simulink model "FSMK_DRC"  (R2015a)
settings: Solver=ode5  StartTime=0.0  StopTime=20  FixedStep=dt  RelTol=1e-3
values from neighbouring files (symbols this model uses):
  A = [0 -87.2734439167 0 0 0 0 87.2734439167 -1.74546887833 0 0 0 0 ... (36 elements, 6x6)]    [A.mat]    (also in A_decompose.m = 0.01*[-0.773996386153021,96.9795539479971,0,0,0,0;-96.400970)
  A_real = A+M_A*N_A*10    [controller.m]
  B = [0  0; 43537  27917; 0  0; 192690  -42273; 0  0; -338240  439030]    [B.mat]    (also in B_decompose.m = 0.01*[-0.230745598618469,-0.153904745996477;0.06127775595526)
  B_real = B+M_B*N_B*10    [controller.m]
  C = [0 -5.1012 0 4.026 0 3.2726]    [C.mat]    (also in C_decompose.m = 0.01*[-23.1554338545303,9.56281796834669,0.435674513053965,-)
  C_real = C+M_C*N_C*10    [controller.m]
  dt = 1e-3    (= 0.001)    [controller.m]
  H = [0 -5.4265 0 5.0795 0 5.0035]    [H.mat]
  Lk = [-59.477792404 31.7484157566 3951.54702126 -4057.82953256 6373.12577438 -2161.86440143]    [Lk.mat]
  Ls = -Ls*1.5e13    [controller.m]
  max_derror = 5    [controller.m]
  max_error = 0.01    [controller.m]
undefined symbols (not defined in the file or in its folder): K
libraries: simulink x2, fuzblock x1
settings Model: Creator=p4wp4w  LastModifiedBy=p4wp4w

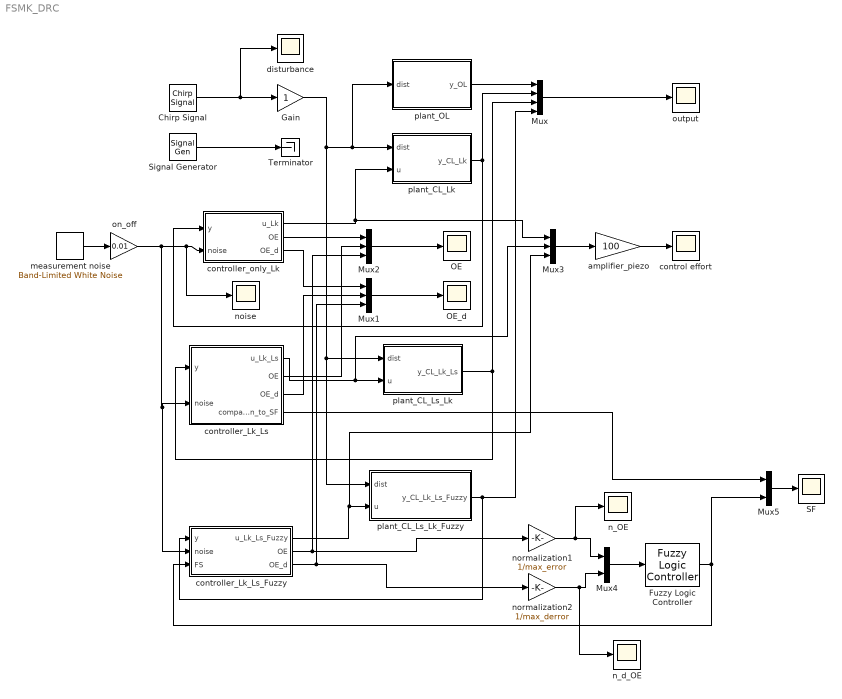
== system FSMK_DRC ==
  Chirp Signal : simulink/Sources/Chirp Signal  f1=0.1  T=20  f2=100
  Fuzzy Logic Controller : fuzblock/Fuzzy Logic  Controller  fis='FSMO.fis'
  Gain : Gain
  Mux : Mux
  Mux1 : Mux  Inputs=3
  Mux2 : Mux  Inputs=3
  Mux3 : Mux  Inputs=3
  Mux4 : Mux  Inputs=2
  Mux5 : Mux  Inputs=2
  OE : Scope
      settings: ShowLegends=on  YMin=-0.01  YMax=0.01  SaveName=OE
  OE_d : Scope
      settings: ShowLegends=on  YMin=-3.5  YMax=3.5  SaveName=d_OE
  SF : Scope
      settings: ShowLegends=on  YMin=-1  YMax=1  SaveName=SF
  Signal Generator : SignalGenerator  WaveForm=square  Frequency=1/5
  Terminator : Terminator
  amplifier_piezo : Gain  Gain=100
  control effort : Scope
      settings: ShowLegends=on  YMin=-50  YMax=50  SaveName=control_effort
  controller_Lk_Ls : Subsystem
  controller_Lk_Ls_Fuzzy : Subsystem
  controller_only_Lk : Subsystem
  disturbance : Scope
      settings: ShowLegends=on  YMin=-1.5  YMax=1.5  SaveName=disturbance
  measurement noise : simulink/Sources/Band-Limited White Noise  Cov=[0.000000001]  Ts=dt  seed=[23341]
  n_OE : Scope
      settings: ShowLegends=on  YMin=-1  YMax=1  SaveName=n_OE
  n_d_OE : Scope
      settings: ShowLegends=on  YMin=-0.8  YMax=0.7  SaveName=n_d_OE
  noise : Scope
      settings: SaveName=ScopeData2
  normalization1 : Gain  Gain=1/max_error
  normalization2 : Gain  Gain=1/max_derror
  on_off : Gain  Gain=0.01
  output : Scope
      settings: ShowLegends=on  YMin=-0.25  YMax=0.25  SaveName=output
  plant_CL_Lk : Subsystem
  plant_CL_Ls_Lk : Subsystem
  plant_CL_Ls_Lk_Fuzzy : Subsystem
  plant_OL : Subsystem
  wires:
  plant_CL_Lk/1(y_CL_Lk) -> controller_only_Lk/1(y), Mux/2
  plant_OL/1(y_OL) -> Mux/1
  controller_only_Lk/1(u_Lk) -> Mux3/1, plant_CL_Lk/2(u)
  measurement noise/1 -> on_off/1
  controller_Lk_Ls/1(u_Lk_Ls) -> Mux3/2, plant_CL_Ls_Lk/2(u)
  controller_only_Lk/3(OE_d) -> Mux1/1
  controller_only_Lk/2(OE) -> Mux2/1
  controller_Lk_Ls/2(OE) -> Mux2/2
  controller_Lk_Ls/3(OE_d) -> Mux1/2
  on_off/1 -> controller_Lk_Ls_Fuzzy/2(noise), controller_Lk_Ls/2(noise), noise/1, controller_only_Lk/2(noise)
  plant_CL_Ls_Lk/1(y_CL_Lk_Ls) -> Mux/3, controller_Lk_Ls/1(y)
  Mux3/1 -> amplifier_piezo/1
  controller_Lk_Ls_Fuzzy/1(u_Lk_Ls_Fuzzy) -> Mux3/3, plant_CL_Ls_Lk_Fuzzy/2(u)
  plant_CL_Ls_Lk_Fuzzy/1(y_CL_Lk_Ls_Fuzzy) -> controller_Lk_Ls_Fuzzy/1(y), Mux/4
  controller_Lk_Ls_Fuzzy/2(OE) -> Mux2/3, normalization1/1
  controller_Lk_Ls_Fuzzy/3(OE_d) -> Mux1/3, normalization2/1
  normalization1/1 -> n_OE/1, Mux4/1
  normalization2/1 -> n_d_OE/1, Mux4/2
  Mux4/1 -> Fuzzy Logic Controller/1
  Fuzzy Logic Controller/1 -> controller_Lk_Ls_Fuzzy/3(FS), Mux5/2
  controller_Lk_Ls/4(comparison_to_SF) -> Mux5/1
  Mux5/1 -> SF/1
  Gain/1 -> plant_CL_Ls_Lk_Fuzzy/1(dist), plant_CL_Ls_Lk/1(dist), plant_OL/1(dist), plant_CL_Lk/1(dist)
  amplifier_piezo/1 -> control effort/1
  Mux/1 -> output/1
  Mux2/1 -> OE/1
  Mux1/1 -> OE_d/1
  Chirp Signal/1 -> disturbance/1, Gain/1
  Signal Generator/1 -> Terminator/1

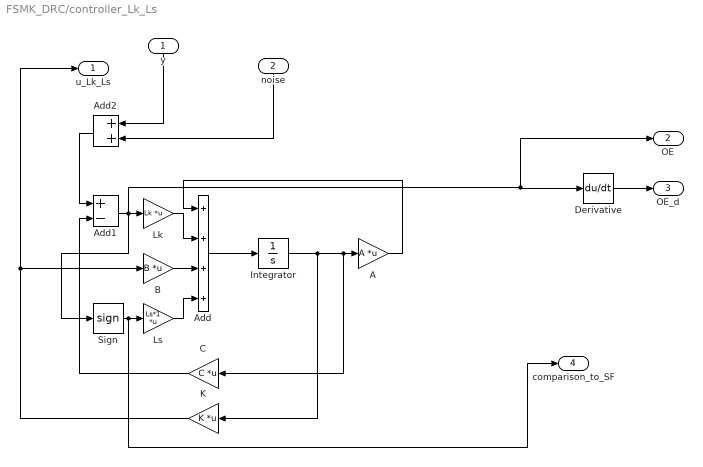
== system FSMK_DRC/controller_Lk_Ls ==
  y : Inport
  noise : Inport  Port=2
  A : Gain  Gain=A  Multiplication=Matrix(K*u)
  Add : Sum  Inputs=++++
  Add1 : Sum  Inputs=+-
  Add2 : Sum
  B : Gain  Gain=B  Multiplication=Matrix(K*u)
  C : Gain  Gain=C  Multiplication=Matrix(K*u)
  Derivative : Derivative
  Integrator : Integrator
  K : Gain  Gain=K  Multiplication=Matrix(K*u)
  Lk : Gain  Gain=Lk  Multiplication=Matrix(K*u)
  Ls : Gain  Gain=Ls*1  Multiplication=Matrix(K*u)
  Sign : Signum
  u_Lk_Ls : Outport
  OE : Outport  Port=2
  OE_d : Outport  Port=3
  comparison_to_SF : Outport  Port=4
  wires:
  Derivative/1 -> OE_d/1
  noise/1 -> Add2/2
  Add1/1 -> Sign/1, Lk/1, OE/1, Derivative/1
  C/1 -> Add1/2
  Add/1 -> Integrator/1
  Add2/1 -> Add1/1
  Lk/1 -> Add/2
  A/1 -> Add/1
  B/1 -> Add/3
  Integrator/1 -> A/1, C/1, K/1
  K/1 -> B/1, u_Lk_Ls/1
  y/1 -> Add2/1
  Ls/1 -> Add/4
  Sign/1 -> comparison_to_SF/1, Ls/1

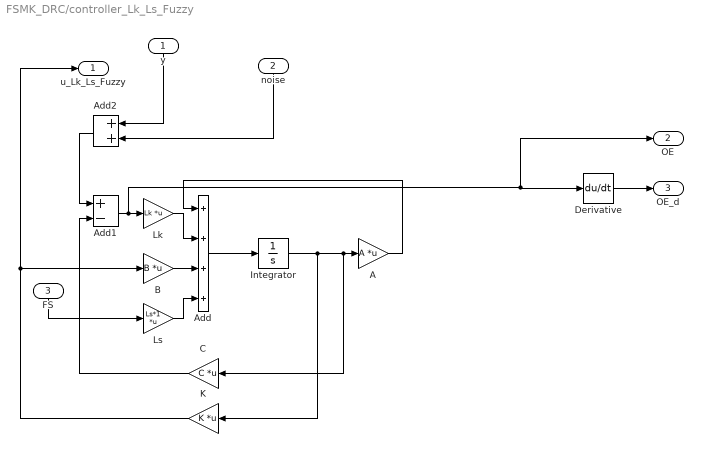
== system FSMK_DRC/controller_Lk_Ls_Fuzzy ==
  y : Inport
  noise : Inport  Port=2
  FS : Inport  Port=3
  A : Gain  Gain=A  Multiplication=Matrix(K*u)
  Add : Sum  Inputs=++++
  Add1 : Sum  Inputs=+-
  Add2 : Sum
  B : Gain  Gain=B  Multiplication=Matrix(K*u)
  C : Gain  Gain=C  Multiplication=Matrix(K*u)
  Derivative : Derivative
  Integrator : Integrator
  K : Gain  Gain=K  Multiplication=Matrix(K*u)
  Lk : Gain  Gain=Lk  Multiplication=Matrix(K*u)
  Ls : Gain  Gain=Ls*1  Multiplication=Matrix(K*u)
  u_Lk_Ls_Fuzzy : Outport
  OE : Outport  Port=2
  OE_d : Outport  Port=3
  wires:
  FS/1 -> Ls/1
  Ls/1 -> Add/4
  y/1 -> Add2/1
  K/1 -> u_Lk_Ls_Fuzzy/1, B/1
  Integrator/1 -> K/1, C/1, A/1
  B/1 -> Add/3
  A/1 -> Add/1
  Lk/1 -> Add/2
  Add2/1 -> Add1/1
  Add/1 -> Integrator/1
  C/1 -> Add1/2
  Add1/1 -> Derivative/1, OE/1, Lk/1
  noise/1 -> Add2/2
  Derivative/1 -> OE_d/1

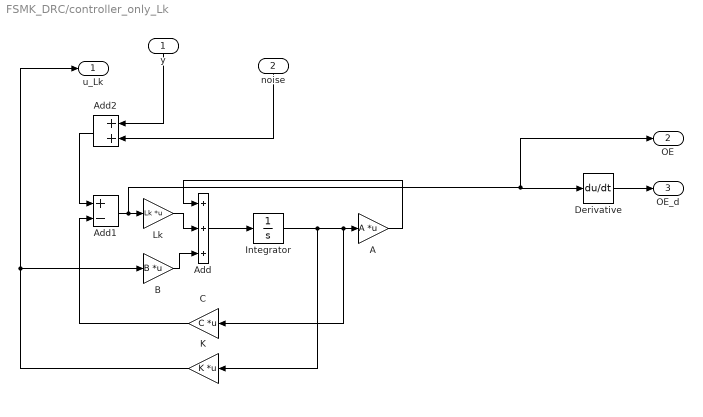
== system FSMK_DRC/controller_only_Lk ==
  y : Inport
  noise : Inport  Port=2
  A : Gain  Gain=A  Multiplication=Matrix(K*u)
  Add : Sum  Inputs=+++
  Add1 : Sum  Inputs=+-
  Add2 : Sum
  B : Gain  Gain=B  Multiplication=Matrix(K*u)
  C : Gain  Gain=C  Multiplication=Matrix(K*u)
  Derivative : Derivative
  Integrator : Integrator
  K : Gain  Gain=K  Multiplication=Matrix(K*u)
  Lk : Gain  Gain=Lk  Multiplication=Matrix(K*u)
  u_Lk : Outport
  OE : Outport  Port=2
  OE_d : Outport  Port=3
  wires:
  y/1 -> Add2/1
  K/1 -> u_Lk/1, B/1
  Integrator/1 -> K/1, C/1, A/1
  B/1 -> Add/3
  A/1 -> Add/1
  Lk/1 -> Add/2
  Add2/1 -> Add1/1
  Add/1 -> Integrator/1
  C/1 -> Add1/2
  Add1/1 -> Derivative/1, OE/1, Lk/1
  noise/1 -> Add2/2
  Derivative/1 -> OE_d/1

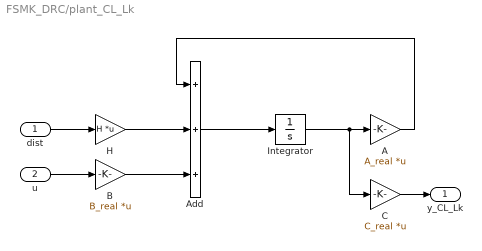
== system FSMK_DRC/plant_CL_Lk ==
  dist : Inport
  u : Inport  Port=2
  A : Gain  Gain=A_real  Multiplication=Matrix(K*u)
  Add : Sum  Inputs=+++
  "B " : Gain  Gain=B_real  Multiplication=Matrix(K*u)
  C : Gain  Gain=C_real  Multiplication=Matrix(K*u)
  H : Gain  Gain=H  Multiplication=Matrix(K*u)
  Integrator : Integrator
  y_CL_Lk : Outport
  wires:
  Add/1 -> Integrator/1
  dist/1 -> H/1
  A/1 -> Add/1
  H/1 -> Add/2
  C/1 -> y_CL_Lk/1
  Integrator/1 -> A/1, C/1
  u/1 -> "B "/1
  "B "/1 -> Add/3

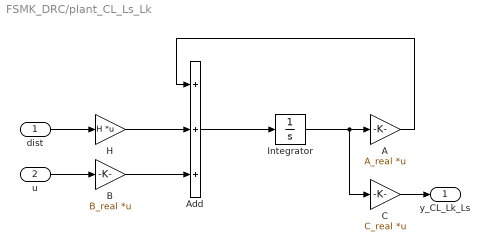
== system FSMK_DRC/plant_CL_Ls_Lk ==
  dist : Inport
  u : Inport  Port=2
  A : Gain  Gain=A_real  Multiplication=Matrix(K*u)
  Add : Sum  Inputs=+++
  "B " : Gain  Gain=B_real  Multiplication=Matrix(K*u)
  C : Gain  Gain=C_real  Multiplication=Matrix(K*u)
  H : Gain  Gain=H  Multiplication=Matrix(K*u)
  Integrator : Integrator
  y_CL_Lk_Ls : Outport
  wires:
  "B "/1 -> Add/3
  u/1 -> "B "/1
  Integrator/1 -> C/1, A/1
  C/1 -> y_CL_Lk_Ls/1
  H/1 -> Add/2
  A/1 -> Add/1
  dist/1 -> H/1
  Add/1 -> Integrator/1

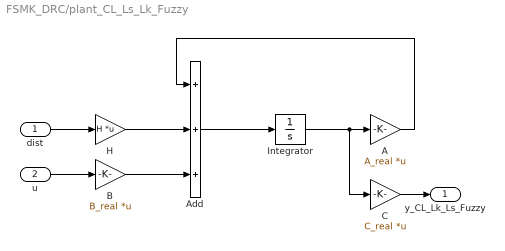
== system FSMK_DRC/plant_CL_Ls_Lk_Fuzzy ==
  dist : Inport
  u : Inport  Port=2
  A : Gain  Gain=A_real  Multiplication=Matrix(K*u)
  Add : Sum  Inputs=+++
  "B " : Gain  Gain=B_real  Multiplication=Matrix(K*u)
  C : Gain  Gain=C_real  Multiplication=Matrix(K*u)
  H : Gain  Gain=H  Multiplication=Matrix(K*u)
  Integrator : Integrator
  y_CL_Lk_Ls_Fuzzy : Outport
  wires:
  Add/1 -> Integrator/1
  dist/1 -> H/1
  A/1 -> Add/1
  H/1 -> Add/2
  C/1 -> y_CL_Lk_Ls_Fuzzy/1
  Integrator/1 -> A/1, C/1
  u/1 -> "B "/1
  "B "/1 -> Add/3

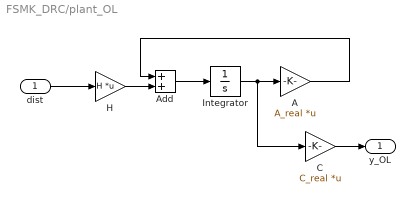
== system FSMK_DRC/plant_OL ==
  dist : Inport
  A : Gain  Gain=A_real  Multiplication=Matrix(K*u)
  Add : Sum
  C : Gain  Gain=C_real  Multiplication=Matrix(K*u)
  H : Gain  Gain=H  Multiplication=Matrix(K*u)
  Integrator : Integrator
  y_OL : Outport
  wires:
  Integrator/1 -> A/1, C/1
  C/1 -> y_OL/1
  H/1 -> Add/2
  A/1 -> Add/1
  dist/1 -> H/1
  Add/1 -> Integrator/1
